simulink model "Tilt_Telescopic_Switch"  (R2022a)
settings: Solver=FixedStepDiscrete  StartTime=0.0  StopTime=inf  FixedStep=0.00001  MaxStep=0.00001  RelTol=1e-3
values from neighbouring files (symbols this model uses):
  k_switchdebounce_time = 50.0    [data_dictionaryy.sldd]
  k_switchrelease_time = 100.0    [data_dictionaryy.sldd]
  k_switchstuck_time = 120.0    [data_dictionaryy.sldd]
  TELE_INPUT : value not decoded    [data_dictionaryy.sldd]
  TILT_INPUT : value not decoded    [data_dictionaryy.sldd]
libraries: simulink x4
settings Model: DataDictionary=data_dictionaryy.sldd  EnableAccessToBaseWorkspace=off  Creator=jamesbond  LastModifiedBy=jamesbond
settings OptimizationCC: BlockReduction=off  DefaultParameterBehavior=Inlined  EnhancedBackFolding=on  PassReuseOutputArgsAs=Individual arguments  ZeroExternalMemoryAtStartup=off  ZeroInternalMemoryAtStartup=off  LifeSpan=inf  OptimizeBlockOrder=speed  DifferentSizesBufferReuse=on  OptimizationCustomize=off  EfficientTunableParamExpr=on
settings DebuggingCC: SignalInfNanChecking=error  ReadBeforeWriteMsg=EnableAllAsError  WriteAfterWriteMsg=EnableAllAsError  WriteAfterReadMsg=EnableAllAsError  AlgebraicLoopMsg=error  ArtificialAlgebraicLoopMsg=error  UnderspecifiedInitializationDetection=Classic  BlockPriorityViolationMsg=error  SolverPrmCheckMsg=warning  InheritedTsInSrcMsg=none  SigSpecEnsureSampleTimeMsg=error  CheckMatrixSingularityMsg=error  IntegerOverflowMsg=error  ParameterPrecisionLossMsg=none  ParameterTunabilityLossMsg=error  UnderSpecifiedDataTypeMsg=error  SignalLabelMismatchMsg=warning  UnconnectedInputMsg=warning  UnconnectedOutputMsg=warning  UnconnectedLineMsg=warning  UniqueDataStoreMsg=error  AssertControl=DisableAll  ModelReferenceIOMsg=error  ModelReferenceIOMismatchMessage=warning  StateNameClashWarn=warning  SFUnexpectedBacktrackingDiag=warning  SFInvalidInputDataAccessInChartInitDiag=error  SFTransitionOutsideNaturalParentDiag=error  SFUndirectedBroadcastEventsDiag=error  SFTransitionActionBeforeConditionDiag=error  IntegerSaturationMsg=error
settings SFSimCC: MATLABDynamicMemAlloc=off
settings RTWCC: SystemTargetFile=ert.tlc  GenCodeOnly=on  TemplateMakefile=ert_default_tmf  GenerateReport=on  GenerateWebview=on
settings CodeAppCC: ForceParamTrailComments=on  IgnoreCustomStorageClasses=off  OperatorAnnotations=on  SimulinkDataObjDesc=on  SFDataObjDesc=on  InsertBlockDesc=on  StateflowObjectComments=on  MATLABSourceComments=on
settings ERTTargetCC: TargetLangStandard=C99 (ISO)  GenerateSampleERTMain=on  SuppressErrorStatus=on  SupportAbsoluteTime=off  SupportNonFinite=off  ParenthesesLevel=Maximum  InlinedParameterPlacement=NonHierarchical  ERTCustomFileTemplate=example_file_process.tlc  PreserveExpressionOrder=on
settings ConfigComp: CovMetricSettings=dcmtrzoiwe

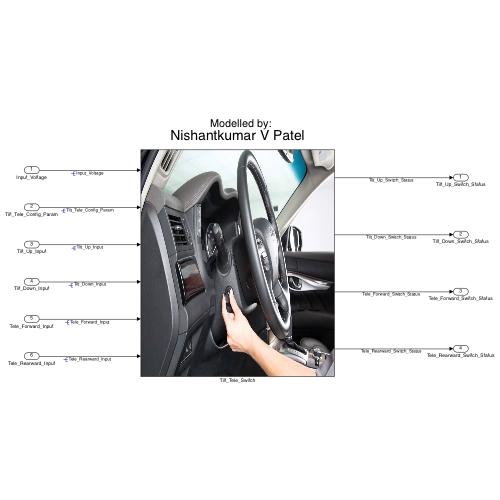
[thumbnail: Simulink's stored preview of the top-level diagram]
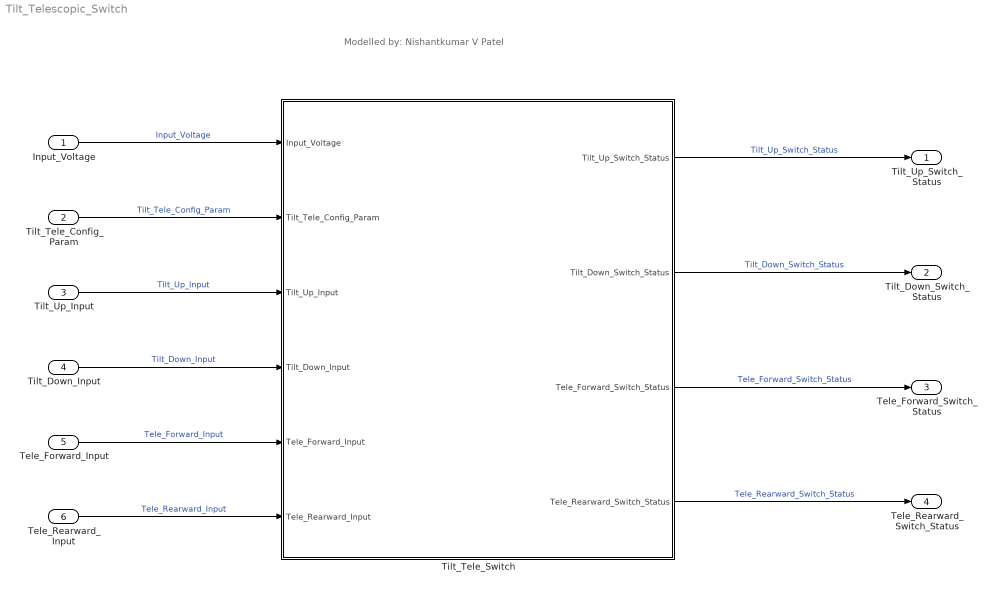
== system Tilt_Telescopic_Switch ==
  note: Modelled by:
      | Nishantkumar V Patel
  Input_Voltage : Inport
  Tilt_Tele_Config_Param : Inport  Port=2
  Tilt_Up_Input : Inport  Port=3
  Tilt_Down_Input : Inport  Port=4
  Tele_Forward_Input : Inport  Port=5
  Tele_Rearward_Input : Inport  Port=6
  Tilt_Tele_Switch : Subsystem
      mask Display: image('$imagefile'); % Use "Edit Image" on toolstrip to change.
  Tilt_Up_Switch_Status : Outport
  Tilt_Down_Switch_Status : Outport  Port=2
  Tele_Forward_Switch_Status : Outport  Port=3
  Tele_Rearward_Switch_Status : Outport  Port=4
  wires:
  Tilt_Tele_Switch/1(Tilt_Up_Switch_Status) -> Tilt_Up_Switch_Status/1  "Tilt_Up_Switch_Status"
  Tilt_Tele_Switch/2(Tilt_Down_Switch_Status) -> Tilt_Down_Switch_Status/1  "Tilt_Down_Switch_Status"
  Tilt_Tele_Switch/3(Tele_Forward_Switch_Status) -> Tele_Forward_Switch_Status/1  "Tele_Forward_Switch_Status"
  Tilt_Tele_Switch/4(Tele_Rearward_Switch_Status) -> Tele_Rearward_Switch_Status/1  "Tele_Rearward_Switch_Status"
  Input_Voltage/1 -> Tilt_Tele_Switch/1(Input_Voltage)  "Input_Voltage"
  Tilt_Tele_Config_Param/1 -> Tilt_Tele_Switch/2(Tilt_Tele_Config_Param)  "Tilt_Tele_Config_Param"
  Tilt_Up_Input/1 -> Tilt_Tele_Switch/3(Tilt_Up_Input)  "Tilt_Up_Input"
  Tilt_Down_Input/1 -> Tilt_Tele_Switch/4(Tilt_Down_Input)  "Tilt_Down_Input"
  Tele_Forward_Input/1 -> Tilt_Tele_Switch/5(Tele_Forward_Input)  "Tele_Forward_Input"
  Tele_Rearward_Input/1 -> Tilt_Tele_Switch/6(Tele_Rearward_Input)  "Tele_Rearward_Input"

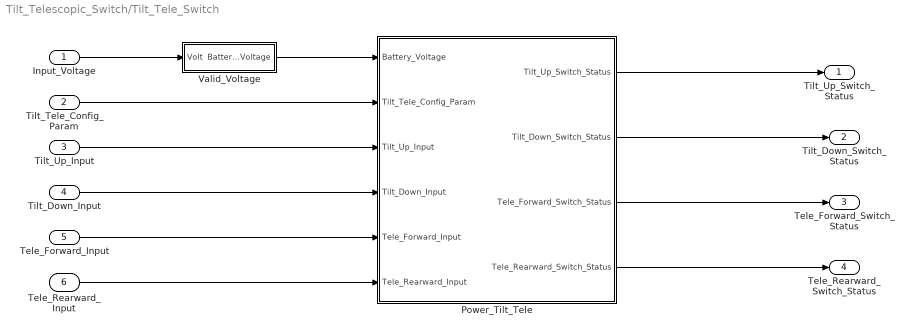
== system Tilt_Telescopic_Switch/Tilt_Tele_Switch ==
  Input_Voltage : Inport
  Tilt_Tele_Config_Param : Inport  Port=2
  Tilt_Up_Input : Inport  Port=3
  Tilt_Down_Input : Inport  Port=4
  Tele_Forward_Input : Inport  Port=5
  Tele_Rearward_Input : Inport  Port=6
  Power_Tilt_Tele : Subsystem
  Valid_Voltage : Subsystem
  Tilt_Up_Switch_Status : Outport
  Tilt_Down_Switch_Status : Outport  Port=2
  Tele_Forward_Switch_Status : Outport  Port=3
  Tele_Rearward_Switch_Status : Outport  Port=4
  wires:
  Input_Voltage/1 -> Valid_Voltage/1(Volt)
  Tilt_Tele_Config_Param/1 -> Power_Tilt_Tele/2(Tilt_Tele_Config_Param)
  Tilt_Up_Input/1 -> Power_Tilt_Tele/3(Tilt_Up_Input)
  Tilt_Down_Input/1 -> Power_Tilt_Tele/4(Tilt_Down_Input)
  Tele_Forward_Input/1 -> Power_Tilt_Tele/5(Tele_Forward_Input)
  Tele_Rearward_Input/1 -> Power_Tilt_Tele/6(Tele_Rearward_Input)
  Valid_Voltage/1(Battery_Voltage) -> Power_Tilt_Tele/1(Battery_Voltage)
  Power_Tilt_Tele/1(Tilt_Up_Switch_Status) -> Tilt_Up_Switch_Status/1
  Power_Tilt_Tele/4(Tele_Rearward_Switch_Status) -> Tele_Rearward_Switch_Status/1
  Power_Tilt_Tele/3(Tele_Forward_Switch_Status) -> Tele_Forward_Switch_Status/1
  Power_Tilt_Tele/2(Tilt_Down_Switch_Status) -> Tilt_Down_Switch_Status/1

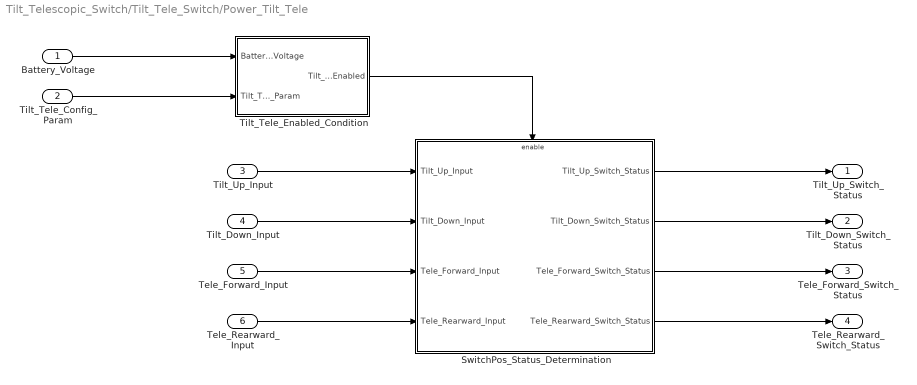
== system Tilt_Telescopic_Switch/Tilt_Tele_Switch/Power_Tilt_Tele ==
  Battery_Voltage : Inport
  Tilt_Tele_Config_Param : Inport  Port=2
  Tilt_Up_Input : Inport  Port=3
  Tilt_Down_Input : Inport  Port=4
  Tele_Forward_Input : Inport  Port=5
  Tele_Rearward_Input : Inport  Port=6
  SwitchPos_Status_Determination : Subsystem  TreatAsAtomicUnit=on
  Tilt_Tele_Enabled_Condition : Subsystem
  Tilt_Up_Switch_Status : Outport
  Tilt_Down_Switch_Status : Outport  Port=2
  Tele_Forward_Switch_Status : Outport  Port=3
  Tele_Rearward_Switch_Status : Outport  Port=4
  wires:
  Tilt_Tele_Config_Param/1 -> Tilt_Tele_Enabled_Condition/2(Tilt_Tele_Config_Param)
  Battery_Voltage/1 -> Tilt_Tele_Enabled_Condition/1(Battery_Voltage)
  Tilt_Tele_Enabled_Condition/1(Tilt_Tele_Enabled) -> SwitchPos_Status_Determination/Enable
  Tilt_Up_Input/1 -> SwitchPos_Status_Determination/1(Tilt_Up_Input)
  Tilt_Down_Input/1 -> SwitchPos_Status_Determination/2(Tilt_Down_Input)
  Tele_Forward_Input/1 -> SwitchPos_Status_Determination/3(Tele_Forward_Input)
  Tele_Rearward_Input/1 -> SwitchPos_Status_Determination/4(Tele_Rearward_Input)
  SwitchPos_Status_Determination/1(Tilt_Up_Switch_Status) -> Tilt_Up_Switch_Status/1
  SwitchPos_Status_Determination/2(Tilt_Down_Switch_Status) -> Tilt_Down_Switch_Status/1
  SwitchPos_Status_Determination/3(Tele_Forward_Switch_Status) -> Tele_Forward_Switch_Status/1
  SwitchPos_Status_Determination/4(Tele_Rearward_Switch_Status) -> Tele_Rearward_Switch_Status/1

== system Tilt_Telescopic_Switch/Tilt_Tele_Switch/Valid_Voltage ==
  Volt : Inport
  Logical Operator : Logic  AllPortsSameDT=off  OutDataTypeStr=boolean
  Relational Operator : RelationalOperator  OutDataTypeStr=boolean  RndMeth=Simplest  InputSameDT=off
  Relational Operator1 : RelationalOperator  Operator=<=  OutDataTypeStr=boolean  RndMeth=Simplest  InputSameDT=off
  VMax : Constant  Value=10
  VMin : Constant  Value=20
  Battery_Voltage : Outport
  wires:
  Volt/1 -> Relational Operator/1, Relational Operator1/1
  VMax/1 -> Relational Operator/2  "VMin"
  VMin/1 -> Relational Operator1/2  "VMax"
  Relational Operator/1 -> Logical Operator/1  "MinVolt"
  Relational Operator1/1 -> Logical Operator/2  "MaxVolt"
  Logical Operator/1 -> Battery_Voltage/1

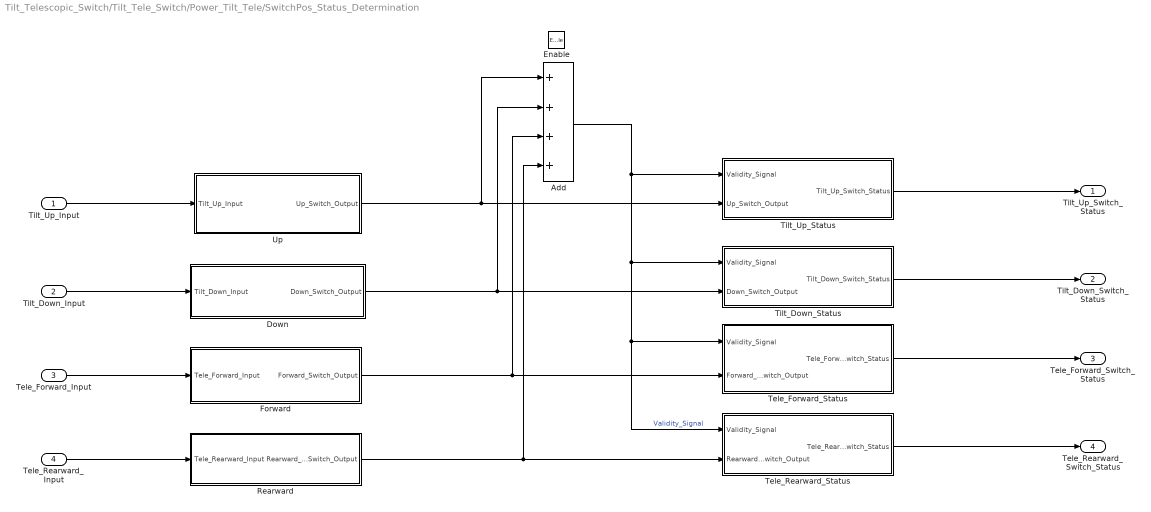
== system Tilt_Telescopic_Switch/Tilt_Tele_Switch/Power_Tilt_Tele/SwitchPos_Status_Determination ==
  Tilt_Up_Input : Inport
  Tilt_Down_Input : Inport  Port=2
  Tele_Forward_Input : Inport  Port=3
  Tele_Rearward_Input : Inport  Port=4
  Enable : EnablePort
  Add : Sum  Inputs=++++
  Down : Subsystem
  Forward : Subsystem
  Rearward : Subsystem
  Tele_Forward_Status : Subsystem
  Tele_Rearward_Status : Subsystem
  Tilt_Down_Status : Subsystem
  Tilt_Up_Status : Subsystem
  Up : Subsystem
  Tilt_Up_Switch_Status : Outport
  Tilt_Down_Switch_Status : Outport  Port=2
  Tele_Forward_Switch_Status : Outport  Port=3
  Tele_Rearward_Switch_Status : Outport  Port=4
  wires:
  Up/1(Up_Switch_Output) -> Add/1, Tilt_Up_Status/2(Up_Switch_Output)
  Down/1(Down_Switch_Output) -> Add/2, Tilt_Down_Status/2(Down_Switch_Output)
  Forward/1(Forward_Switch_Output) -> Add/3, Tele_Forward_Status/2(Forward_Switch_Output)
  Rearward/1(Rearward_Switch_Output) -> Add/4, Tele_Rearward_Status/2(Rearward_Switch_Output)
  Tilt_Up_Input/1 -> Up/1(Tilt_Up_Input)
  Tilt_Down_Input/1 -> Down/1(Tilt_Down_Input)
  Tele_Forward_Input/1 -> Forward/1(Tele_Forward_Input)
  Tele_Rearward_Input/1 -> Rearward/1(Tele_Rearward_Input)
  Add/1 -> Tele_Rearward_Status/1(Validity_Signal), Tele_Forward_Status/1(Validity_Signal), Tilt_Down_Status/1(Validity_Signal), Tilt_Up_Status/1(Validity_Signal)  "Validity_Signal"
  Tilt_Up_Status/1(Tilt_Up_Switch_Status) -> Tilt_Up_Switch_Status/1
  Tilt_Down_Status/1(Tilt_Down_Switch_Status) -> Tilt_Down_Switch_Status/1
  Tele_Forward_Status/1(Tele_Forward_Switch_Status) -> Tele_Forward_Switch_Status/1
  Tele_Rearward_Status/1(Tele_Rearward_Switch_Status) -> Tele_Rearward_Switch_Status/1

== system Tilt_Telescopic_Switch/Tilt_Tele_Switch/Power_Tilt_Tele/Tilt_Tele_Enabled_Condition ==
  Battery_Voltage : Inport
  Tilt_Tele_Config_Param : Inport  Port=2
  Logical Operator : Logic  AllPortsSameDT=off  OutDataTypeStr=boolean
  Tilt_Tele_Enabled : Outport
  wires:
  Battery_Voltage/1 -> Logical Operator/1
  Tilt_Tele_Config_Param/1 -> Logical Operator/2
  Logical Operator/1 -> Tilt_Tele_Enabled/1  "Tilt_Tele_Enabled"

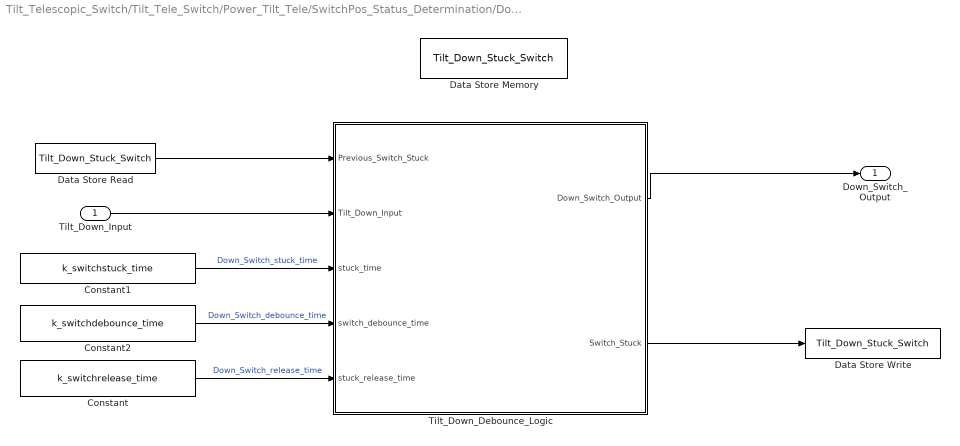
== system Tilt_Telescopic_Switch/Tilt_Tele_Switch/Power_Tilt_Tele/SwitchPos_Status_Determination/Down ==
  Tilt_Down_Input : Inport
  Constant : Constant  Value=k_switchrelease_time
  Constant1 : Constant  Value=k_switchstuck_time
  Constant2 : Constant  Value=k_switchdebounce_time
  Data Store Memory : DataStoreMemory  DataStoreName=Tilt_Down_Stuck_Switch  WriteAfterWriteMsg=warning  ShowAdditionalParam=off  StateMustResolveToSignalObject=on
  Data Store Read : DataStoreRead  DataStoreName=Tilt_Down_Stuck_Switch  IndexOptions=Index vector (dialog)  Indices=1  OutputSizes=1
  Data Store Write : DataStoreWrite  DataStoreName=Tilt_Down_Stuck_Switch  IndexOptions=Index vector (dialog)  Indices=1  OutputSizes=1
  Tilt_Down_Debounce_Logic : Stateflow chart  TreatAsAtomicUnit=on
  Down_Switch_Output : Outport
  wires:
  Data Store Read/1 -> Tilt_Down_Debounce_Logic/1(Previous_Switch_Stuck)
  Tilt_Down_Debounce_Logic/2(Switch_Stuck) -> Data Store Write/1
  Tilt_Down_Input/1 -> Tilt_Down_Debounce_Logic/2(Tilt_Down_Input)
  Tilt_Down_Debounce_Logic/1(Down_Switch_Output) -> Down_Switch_Output/1
  Constant/1 -> Tilt_Down_Debounce_Logic/5(stuck_release_time)  "Down_Switch_release_time"
  Constant2/1 -> Tilt_Down_Debounce_Logic/4(switch_debounce_time)  "Down_Switch_debounce_time"
  Constant1/1 -> Tilt_Down_Debounce_Logic/3(stuck_time)  "Down_Switch_stuck_time"

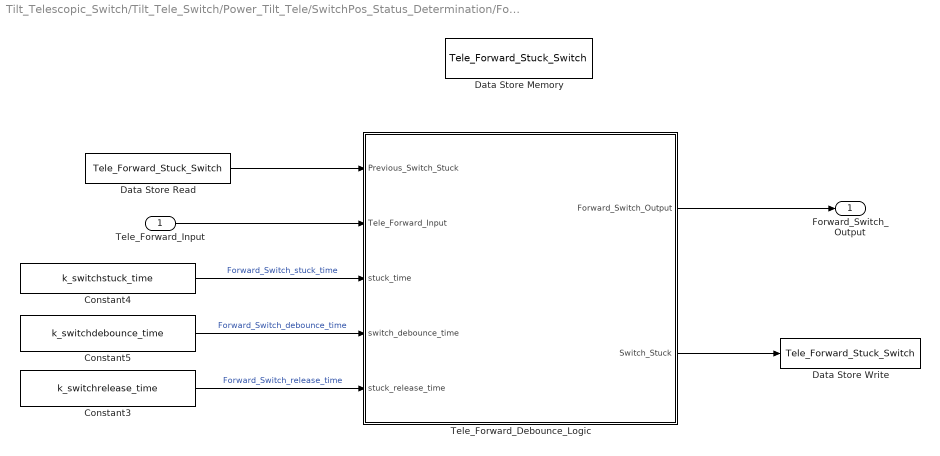
== system Tilt_Telescopic_Switch/Tilt_Tele_Switch/Power_Tilt_Tele/SwitchPos_Status_Determination/Forward ==
  Tele_Forward_Input : Inport
  Constant3 : Constant  Value=k_switchrelease_time
  Constant4 : Constant  Value=k_switchstuck_time
  Constant5 : Constant  Value=k_switchdebounce_time
  Data Store Memory : DataStoreMemory  DataStoreName=Tele_Forward_Stuck_Switch  WriteAfterWriteMsg=warning  ShowAdditionalParam=off  StateMustResolveToSignalObject=on
  Data Store Read : DataStoreRead  DataStoreName=Tele_Forward_Stuck_Switch  IndexOptions=Index vector (dialog)  Indices=1  OutputSizes=1
  Data Store Write : DataStoreWrite  DataStoreName=Tele_Forward_Stuck_Switch  IndexOptions=Index vector (dialog)  Indices=1  OutputSizes=1
  Tele_Forward_Debounce_Logic : Stateflow chart  TreatAsAtomicUnit=on
  Forward_Switch_Output : Outport
  wires:
  Constant4/1 -> Tele_Forward_Debounce_Logic/3(stuck_time)  "Forward_Switch_stuck_time"
  Tele_Forward_Input/1 -> Tele_Forward_Debounce_Logic/2(Tele_Forward_Input)
  Constant5/1 -> Tele_Forward_Debounce_Logic/4(switch_debounce_time)  "Forward_Switch_debounce_time"
  Data Store Read/1 -> Tele_Forward_Debounce_Logic/1(Previous_Switch_Stuck)
  Tele_Forward_Debounce_Logic/2(Switch_Stuck) -> Data Store Write/1
  Tele_Forward_Debounce_Logic/1(Forward_Switch_Output) -> Forward_Switch_Output/1
  Constant3/1 -> Tele_Forward_Debounce_Logic/5(stuck_release_time)  "Forward_Switch_release_time"

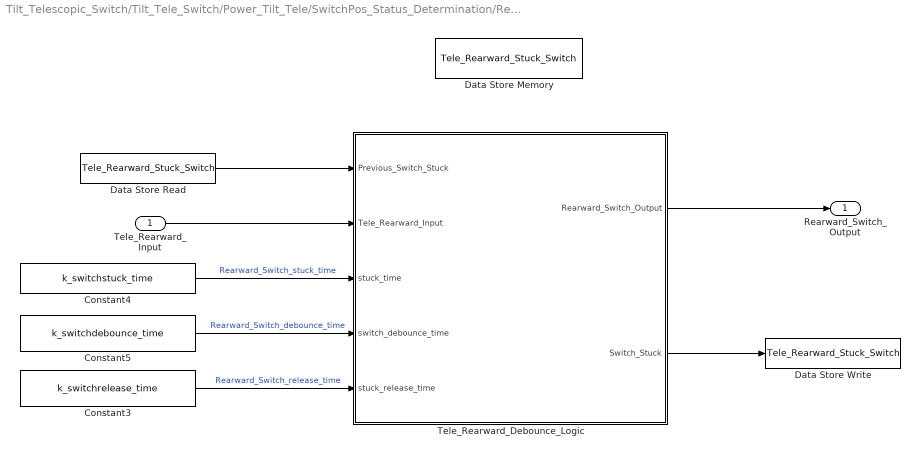
== system Tilt_Telescopic_Switch/Tilt_Tele_Switch/Power_Tilt_Tele/SwitchPos_Status_Determination/Rearward ==
  Tele_Rearward_Input : Inport
  Constant3 : Constant  Value=k_switchrelease_time
  Constant4 : Constant  Value=k_switchstuck_time
  Constant5 : Constant  Value=k_switchdebounce_time
  Data Store Memory : DataStoreMemory  DataStoreName=Tele_Rearward_Stuck_Switch  WriteAfterWriteMsg=warning  ShowAdditionalParam=off  StateMustResolveToSignalObject=on
  Data Store Read : DataStoreRead  DataStoreName=Tele_Rearward_Stuck_Switch  IndexOptions=Index vector (dialog)  Indices=1  OutputSizes=1
  Data Store Write : DataStoreWrite  DataStoreName=Tele_Rearward_Stuck_Switch  IndexOptions=Index vector (dialog)  Indices=1  OutputSizes=1
  Tele_Rearward_Debounce_Logic : Stateflow chart  TreatAsAtomicUnit=on
  Rearward_Switch_Output : Outport
  wires:
  Constant4/1 -> Tele_Rearward_Debounce_Logic/3(stuck_time)  "Rearward_Switch_stuck_time"
  Tele_Rearward_Input/1 -> Tele_Rearward_Debounce_Logic/2(Tele_Rearward_Input)
  Constant5/1 -> Tele_Rearward_Debounce_Logic/4(switch_debounce_time)  "Rearward_Switch_debounce_time"
  Data Store Read/1 -> Tele_Rearward_Debounce_Logic/1(Previous_Switch_Stuck)
  Tele_Rearward_Debounce_Logic/2(Switch_Stuck) -> Data Store Write/1
  Tele_Rearward_Debounce_Logic/1(Rearward_Switch_Output) -> Rearward_Switch_Output/1
  Constant3/1 -> Tele_Rearward_Debounce_Logic/5(stuck_release_time)  "Rearward_Switch_release_time"

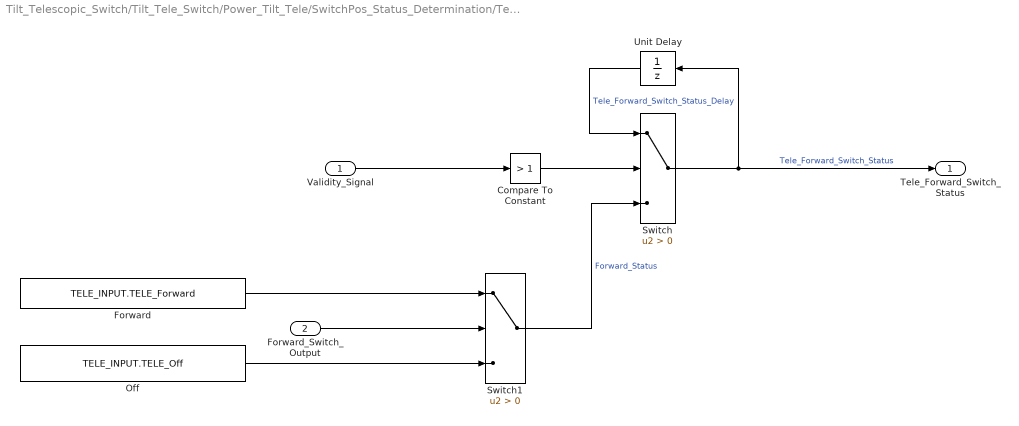
== system Tilt_Telescopic_Switch/Tilt_Tele_Switch/Power_Tilt_Tele/SwitchPos_Status_Determination/Tele_Forward_Status ==
  Validity_Signal : Inport
  Forward_Switch_Output : Inport  Port=2
  Compare To Constant : simulink/Logic and Bit Operations/Compare To Constant  relop=>  const=1  OutDataTypeStr=boolean
  Forward : Constant  Value=TELE_INPUT.TELE_Forward
  Off : Constant  Value=TELE_INPUT.TELE_Off
  Switch : Switch  Criteria=u2 > Threshold  SaturateOnIntegerOverflow=off  InputSameDT=off
  Switch1 : Switch  Criteria=u2 > Threshold  SaturateOnIntegerOverflow=off  InputSameDT=off
  Unit Delay : UnitDelay  InitialCondition=TELE_INPUT.TELE_Off  SampleTime=-1  StateName=Tele_Forward_Switch_Status_Delay  HasFrameUpgradeWarning=on  StateMustResolveToSignalObject=on
  Tele_Forward_Switch_Status : Outport
  wires:
  Switch1/1 -> Switch/3  "Forward_Status"
  Switch/1 -> Tele_Forward_Switch_Status/1, Unit Delay/1  "Tele_Forward_Switch_Status"
  Forward/1 -> Switch1/1
  Off/1 -> Switch1/3
  Compare To Constant/1 -> Switch/2
  Forward_Switch_Output/1 -> Switch1/2
  Unit Delay/1 -> Switch/1  "Tele_Forward_Switch_Status_Delay"
  Validity_Signal/1 -> Compare To Constant/1

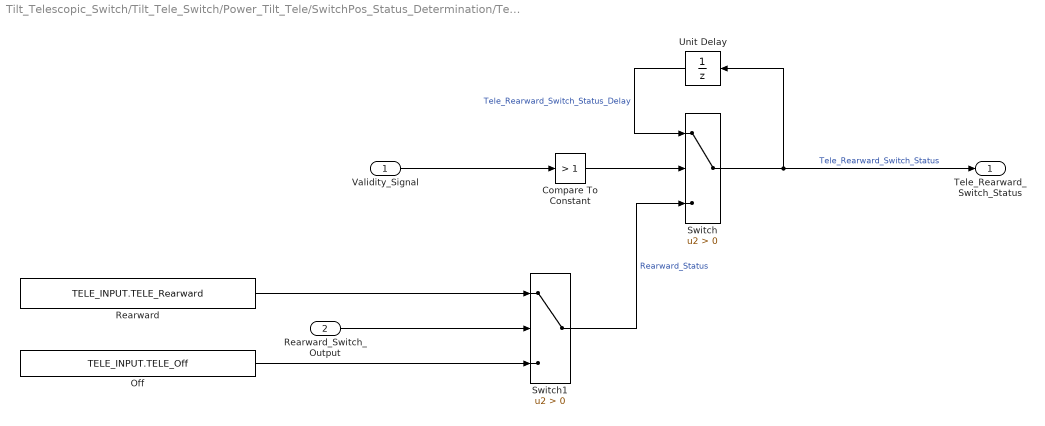
== system Tilt_Telescopic_Switch/Tilt_Tele_Switch/Power_Tilt_Tele/SwitchPos_Status_Determination/Tele_Rearward_Status ==
  Validity_Signal : Inport
  Rearward_Switch_Output : Inport  Port=2
  Compare To Constant : simulink/Logic and Bit Operations/Compare To Constant  relop=>  const=1  OutDataTypeStr=boolean
  Off : Constant  Value=TELE_INPUT.TELE_Off
  Rearward : Constant  Value=TELE_INPUT.TELE_Rearward
  Switch : Switch  Criteria=u2 > Threshold  SaturateOnIntegerOverflow=off  InputSameDT=off
  Switch1 : Switch  Criteria=u2 > Threshold  SaturateOnIntegerOverflow=off  InputSameDT=off
  Unit Delay : UnitDelay  InitialCondition=TELE_INPUT.TELE_Off  SampleTime=-1  StateName=Tele_Rearward_Switch_Status_Delay  HasFrameUpgradeWarning=on  StateMustResolveToSignalObject=on
  Tele_Rearward_Switch_Status : Outport
  wires:
  Rearward_Switch_Output/1 -> Switch1/2
  Compare To Constant/1 -> Switch/2
  Switch/1 -> Tele_Rearward_Switch_Status/1, Unit Delay/1  "Tele_Rearward_Switch_Status"
  Rearward/1 -> Switch1/1
  Off/1 -> Switch1/3
  Switch1/1 -> Switch/3  "Rearward_Status"
  Unit Delay/1 -> Switch/1  "Tele_Rearward_Switch_Status_Delay"
  Validity_Signal/1 -> Compare To Constant/1

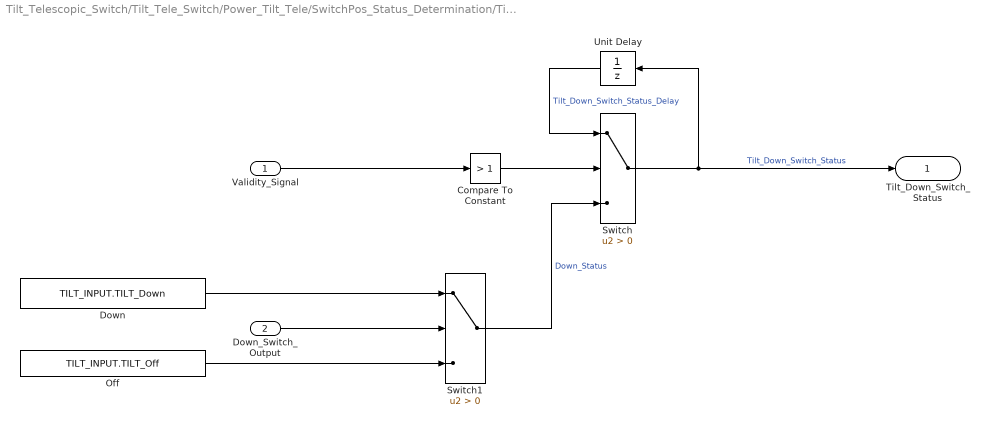
== system Tilt_Telescopic_Switch/Tilt_Tele_Switch/Power_Tilt_Tele/SwitchPos_Status_Determination/Tilt_Down_Status ==
  Validity_Signal : Inport
  Down_Switch_Output : Inport  Port=2
  Compare To Constant : simulink/Logic and Bit Operations/Compare To Constant  relop=>  const=1  OutDataTypeStr=boolean
  Down : Constant  Value=TILT_INPUT.TILT_Down
  Off : Constant  Value=TILT_INPUT.TILT_Off
  Switch : Switch  Criteria=u2 > Threshold  SaturateOnIntegerOverflow=off  InputSameDT=off
  Switch1 : Switch  Criteria=u2 > Threshold  SaturateOnIntegerOverflow=off  InputSameDT=off
  Unit Delay : UnitDelay  InitialCondition=TILT_INPUT.TILT_Off  SampleTime=-1  StateName=Tilt_Down_Switch_Status_Delay  HasFrameUpgradeWarning=on  StateMustResolveToSignalObject=on
  Tilt_Down_Switch_Status : Outport
  wires:
  Off/1 -> Switch1/3
  Compare To Constant/1 -> Switch/2
  Switch1/1 -> Switch/3  "Down_Status"
  Unit Delay/1 -> Switch/1  "Tilt_Down_Switch_Status_Delay"
  Down/1 -> Switch1/1
  Switch/1 -> Unit Delay/1, Tilt_Down_Switch_Status/1  "Tilt_Down_Switch_Status"
  Validity_Signal/1 -> Compare To Constant/1
  Down_Switch_Output/1 -> Switch1/2

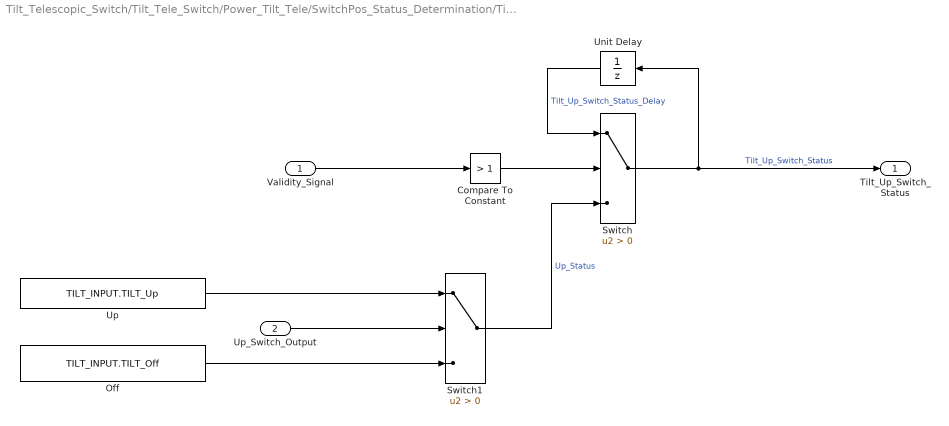
== system Tilt_Telescopic_Switch/Tilt_Tele_Switch/Power_Tilt_Tele/SwitchPos_Status_Determination/Tilt_Up_Status ==
  Validity_Signal : Inport
  Up_Switch_Output : Inport  Port=2
  Compare To Constant : simulink/Logic and Bit Operations/Compare To Constant  relop=>  const=1  OutDataTypeStr=boolean
  Off : Constant  Value=TILT_INPUT.TILT_Off
  Switch : Switch  Criteria=u2 > Threshold  SaturateOnIntegerOverflow=off  InputSameDT=off
  Switch1 : Switch  Criteria=u2 > Threshold  SaturateOnIntegerOverflow=off  InputSameDT=off
  Unit Delay : UnitDelay  InitialCondition=TILT_INPUT.TILT_Off  SampleTime=-1  StateName=Tilt_Up_Switch_Status_Delay  HasFrameUpgradeWarning=on  StateMustResolveToSignalObject=on
  Up : Constant  Value=TILT_INPUT.TILT_Up
  Tilt_Up_Switch_Status : Outport
  wires:
  Compare To Constant/1 -> Switch/2
  Validity_Signal/1 -> Compare To Constant/1
  Switch/1 -> Unit Delay/1, Tilt_Up_Switch_Status/1  "Tilt_Up_Switch_Status"
  Switch1/1 -> Switch/3  "Up_Status"
  Up_Switch_Output/1 -> Switch1/2
  Up/1 -> Switch1/1
  Off/1 -> Switch1/3
  Unit Delay/1 -> Switch/1  "Tilt_Up_Switch_Status_Delay"

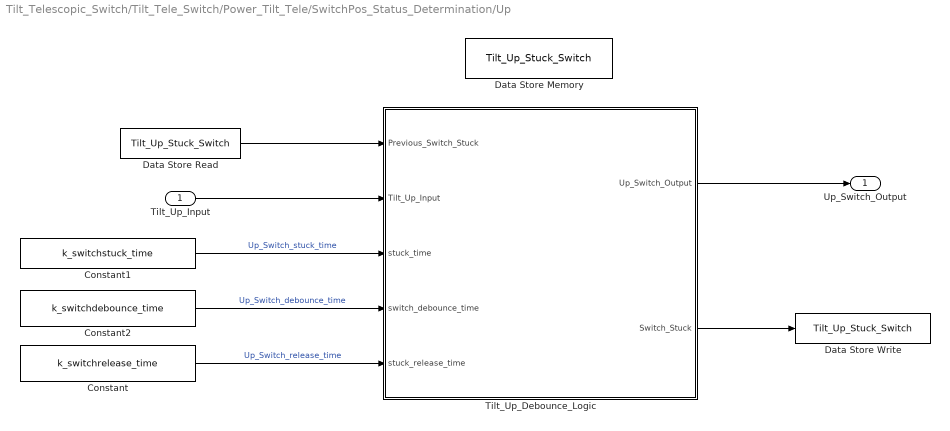
== system Tilt_Telescopic_Switch/Tilt_Tele_Switch/Power_Tilt_Tele/SwitchPos_Status_Determination/Up ==
  Tilt_Up_Input : Inport
  Constant : Constant  Value=k_switchrelease_time
  Constant1 : Constant  Value=k_switchstuck_time
  Constant2 : Constant  Value=k_switchdebounce_time
  Data Store Memory : DataStoreMemory  DataStoreName=Tilt_Up_Stuck_Switch  WriteAfterWriteMsg=warning  ShowAdditionalParam=off  StateMustResolveToSignalObject=on
  Data Store Read : DataStoreRead  DataStoreName=Tilt_Up_Stuck_Switch  IndexOptions=Index vector (dialog)  Indices=1  OutputSizes=1
  Data Store Write : DataStoreWrite  DataStoreName=Tilt_Up_Stuck_Switch  IndexOptions=Index vector (dialog)  Indices=1  OutputSizes=1
  Tilt_Up_Debounce_Logic : Stateflow chart  TreatAsAtomicUnit=on
  Up_Switch_Output : Outport
  wires:
  Constant1/1 -> Tilt_Up_Debounce_Logic/3(stuck_time)  "Up_Switch_stuck_time"
  Constant2/1 -> Tilt_Up_Debounce_Logic/4(switch_debounce_time)  "Up_Switch_debounce_time"
  Tilt_Up_Input/1 -> Tilt_Up_Debounce_Logic/2(Tilt_Up_Input)
  Tilt_Up_Debounce_Logic/1(Up_Switch_Output) -> Up_Switch_Output/1
  Tilt_Up_Debounce_Logic/2(Switch_Stuck) -> Data Store Write/1
  Data Store Read/1 -> Tilt_Up_Debounce_Logic/1(Previous_Switch_Stuck)
  Constant/1 -> Tilt_Up_Debounce_Logic/5(stuck_release_time)  "Up_Switch_release_time"

== stateflow chart Tilt_Telescopic_Switch/Tilt_Tele_Switch/Power_Tilt_Tele/SwitchPos_Status_Determination/Rearward/Tele_Rearward_Debounce_Logic ==
  state Not_Pressed
    en:
    Rearward_Switch_Output = false;
  state Debounce
    state Off_Debounce
    state On_Debounce
  state Off
  state Pressed
    en:
    Rearward_Switch_Output= true;
  state Stuck_Wait
  state Stuck
    en:
    Rearward_Switch_Output= false;
    Switch_Stuck= true;
  (default) -> Not_Pressed
  Off -> Not_Pressed : [after(stuck_release_time,sec)]
  Not_Pressed -> On_Debounce : [(Previous_Switch_Stuck== false)&&(Tele_Rearward_Input==true)]
  Pressed -> Off_Debounce [order 2]
  On_Debounce -> Pressed : [after(switch_debounce_time,sec)]
  Stuck -> Off : [Tele_Rearward_Input==false]
  Pressed -> Stuck_Wait [order 1] : [after(stuck_time-switch_debounce_time,sec)]
  Stuck_Wait -> Stuck : [Tele_Rearward_Input==true]
  data: Previous_Switch_Stuck input boolean; Tele_Rearward_Input input boolean; stuck_time input uint8; switch_debounce_time input uint8; Rearward_Switch_Output output boolean; Switch_Stuck output boolean; stuck_release_time input uint8

== stateflow chart Tilt_Telescopic_Switch/Tilt_Tele_Switch/Power_Tilt_Tele/SwitchPos_Status_Determination/Down/Tilt_Down_Debounce_Logic ==
  state Not_Pressed
    en:
    Down_Switch_Output = false;
  state Debounce
    state Off_Debounce
    state On_Debounce
  state Off
  state Pressed
    en:
    Down_Switch_Output= true;
  state Stuck_Wait
  state Stuck
    en:
    Down_Switch_Output= false;
    Switch_Stuck= true;
  (default) -> Not_Pressed
  Off -> Not_Pressed : [after(stuck_release_time,sec)]
  Not_Pressed -> On_Debounce : [(Previous_Switch_Stuck== false)&&(Tilt_Down_Input==true)]
  Pressed -> Off_Debounce [order 2]
  On_Debounce -> Pressed : [after(switch_debounce_time,sec)]
  Stuck -> Off : [Tilt_Down_Input==false]
  Pressed -> Stuck_Wait [order 1] : [after(stuck_time-switch_debounce_time,sec)]
  Stuck_Wait -> Stuck : [Tilt_Down_Input==true]
  data: Previous_Switch_Stuck input boolean; Tilt_Down_Input input boolean; stuck_time input uint8; switch_debounce_time input uint8; Down_Switch_Output output boolean; Switch_Stuck output boolean; stuck_release_time input uint8

== stateflow chart Tilt_Telescopic_Switch/Tilt_Tele_Switch/Power_Tilt_Tele/SwitchPos_Status_Determination/Forward/Tele_Forward_Debounce_Logic ==
  state Not_Pressed
    en:
    Forward_Switch_Output = false;
  state Debounce
    state Off_Debounce
    state On_Debounce
  state Off
  state Pressed
    en:
    Forward_Switch_Output= true;
  state Stuck_Wait
  state Stuck
    en:
    Forward_Switch_Output= false;
    Switch_Stuck= true;
  (default) -> Not_Pressed
  Off -> Not_Pressed : [after(stuck_release_time,sec)]
  Not_Pressed -> On_Debounce : [(Previous_Switch_Stuck== false)&&(Tele_Forward_Input==true)]
  Pressed -> Off_Debounce [order 2]
  On_Debounce -> Pressed : [after(switch_debounce_time,sec)]
  Stuck -> Off : [Tele_Forward_Input==false]
  Pressed -> Stuck_Wait [order 1] : [after(stuck_time-switch_debounce_time,sec)]
  Stuck_Wait -> Stuck : [Tele_Forward_Input==true]
  data: Previous_Switch_Stuck input boolean; Tele_Forward_Input input boolean; stuck_time input uint8; switch_debounce_time input uint8; Forward_Switch_Output output boolean; Switch_Stuck output boolean; stuck_release_time input uint8

== stateflow chart Tilt_Telescopic_Switch/Tilt_Tele_Switch/Power_Tilt_Tele/SwitchPos_Status_Determination/Up/Tilt_Up_Debounce_Logic ==
  state Not_Pressed
    en:
    Up_Switch_Output = false;
  state Debounce
    state Off_Debounce
    state On_Debounce
  state Off
  state Pressed
    en:
    Up_Switch_Output= true;
  state Stuck_Wait
  state Stuck
    en:
    Up_Switch_Output= false;
    Switch_Stuck= true;
  (default) -> Not_Pressed
  Off -> Not_Pressed : [after(stuck_release_time,sec)]
  Not_Pressed -> On_Debounce : [(Previous_Switch_Stuck== false)&&(Tilt_Up_Input==true)]
  Pressed -> Off_Debounce [order 2]
  On_Debounce -> Pressed : [after(switch_debounce_time,sec)]
  Stuck -> Off : [Tilt_Up_Input==false]
  Pressed -> Stuck_Wait [order 1] : [after(stuck_time-switch_debounce_time,sec)]
  Stuck_Wait -> Stuck : [Tilt_Up_Input==true]
  data: Previous_Switch_Stuck input boolean; Tilt_Up_Input input boolean; stuck_time input uint8; switch_debounce_time input uint8; Up_Switch_Output output boolean; Switch_Stuck output boolean; stuck_release_time input uint8
